simulink model "Verification_Decision_Module_w_History"  (R2015a)
settings: Solver=FixedStepDiscrete  StartTime=0.0  StopTime=10.0  FixedStep=delta_t  RelTol=1e-3
libraries: sldvlib x16
settings Model: Creator=Kerianne  LastModifiedBy=Kerianne
settings DataIOCC: SaveFormat=Structure
settings OptimizationCC: InlineParams=on  ExpressionDepthLimit=2147483647
settings DebuggingCC: UnderspecifiedInitializationDetection=Classic  MergeDetectMultiDrivingBlocksExec=none  SolverPrmCheckMsg=warning  StateNameClashWarn=warning
settings ConfigComp: Description=Design Verifier Custom Configuration Component  DVMaxTestCaseSteps=500  DVTestSuiteOptimization=CombinedObjectives (Nonlinear Extended)

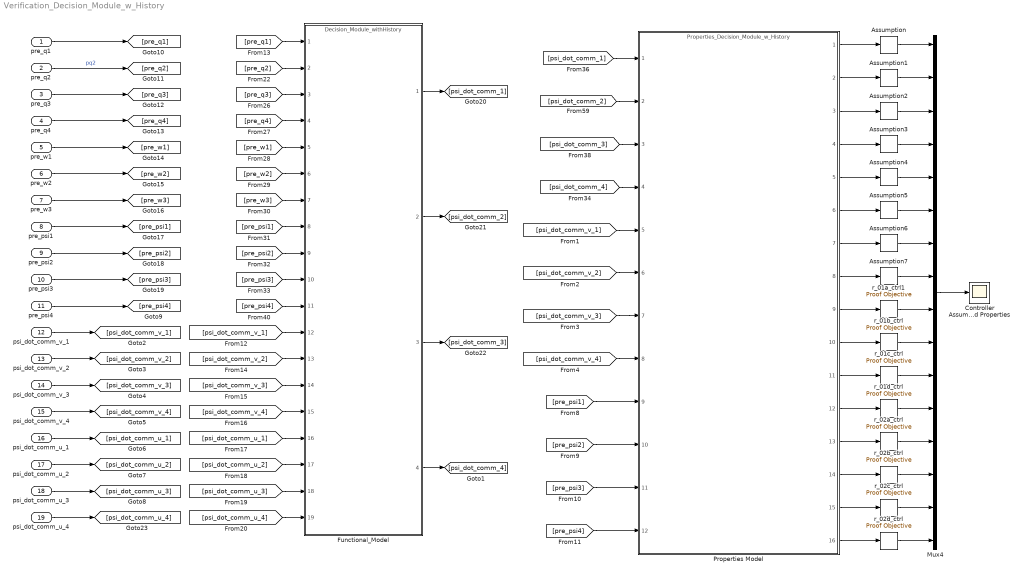
== system Verification_Decision_Module_w_History ==
  pre_q1 : Inport
  pre_q2 : Inport  Port=2
  pre_q3 : Inport  Port=3
  pre_q4 : Inport  Port=4
  pre_w1 : Inport  Port=5
  pre_w2 : Inport  Port=6
  pre_w3 : Inport  Port=7
  pre_psi1 : Inport  Port=8
  pre_psi2 : Inport  Port=9
  pre_psi3 : Inport  Port=10
  pre_psi4 : Inport  Port=11
  psi_dot_comm_v_1 : Inport  Port=12
  psi_dot_comm_v_2 : Inport  Port=13
  psi_dot_comm_v_3 : Inport  Port=14
  psi_dot_comm_v_4 : Inport  Port=15
  psi_dot_comm_u_1 : Inport  Port=16
  psi_dot_comm_u_2 : Inport  Port=17
  psi_dot_comm_u_3 : Inport  Port=18
  psi_dot_comm_u_4 : Inport  Port=19
  Assumption{,1..7} (8 alike) : sldvlib/Objectives and Constraints/Assumption  enabled=on  customAVTBlockType=Assumption  intervals=true  initial=off  dispValues=on  outEnabled=on
      settings: AttributesFormatString=%<intervals>
  Controller Assumptions and Properties : Scope
      settings: ShowLegends=on  YMin=-1  YMax=2
  Functional_Model : ModelReference  ModelNameDialog=Decision_Module_withHistory.slx  SimulationMode=Normal  ModelReferenceVersion=1.60  CopyOfModelName=Decision_Module_withHistory.slx  DefaultDataLogging=on
  Mux4 : Mux  Inputs=16
  Properties Model : ModelReference  ModelNameDialog=Properties_Decision_Module_w_History.slx  SimulationMode=Normal  ModelReferenceVersion=1.94  CopyOfModelName=Properties_Decision_Module_w_History.slx  DefaultDataLogging=on
  r_01a_ctrl1 : sldvlib/Objectives and Constraints/Proof Objective  Tag=g4  enabled=on  customAVTBlockType=Proof Objective  intervals=true  dispValues=on  outEnabled=on  enableStopSim=off
      settings: AttributesFormatString=%<intervals>
  r_01b_ctrl : sldvlib/Objectives and Constraints/Proof Objective  Tag=g4  enabled=on  customAVTBlockType=Proof Objective  intervals=true  dispValues=on  outEnabled=on  enableStopSim=off
      settings: AttributesFormatString=%<intervals>
  r_01c_ctrl : sldvlib/Objectives and Constraints/Proof Objective  Tag=g4  enabled=on  customAVTBlockType=Proof Objective  intervals=true  dispValues=on  outEnabled=on  enableStopSim=off
      settings: AttributesFormatString=%<intervals>
  r_01d_ctrl : sldvlib/Objectives and Constraints/Proof Objective  Tag=g4  enabled=on  customAVTBlockType=Proof Objective  intervals=true  dispValues=on  outEnabled=on  enableStopSim=off
      settings: AttributesFormatString=%<intervals>
  r_02a_ctrl : sldvlib/Objectives and Constraints/Proof Objective  Tag=g4  enabled=on  customAVTBlockType=Proof Objective  intervals=true  dispValues=on  outEnabled=on  enableStopSim=off
      settings: AttributesFormatString=%<intervals>
  r_02b_ctrl : sldvlib/Objectives and Constraints/Proof Objective  Tag=g4  enabled=on  customAVTBlockType=Proof Objective  intervals=true  dispValues=on  outEnabled=on  enableStopSim=off
      settings: AttributesFormatString=%<intervals>
  r_02c_ctrl : sldvlib/Objectives and Constraints/Proof Objective  Tag=g4  enabled=on  customAVTBlockType=Proof Objective  intervals=true  dispValues=on  outEnabled=on  enableStopSim=off
      settings: AttributesFormatString=%<intervals>
  r_02d_ctrl : sldvlib/Objectives and Constraints/Proof Objective  Tag=g4  enabled=on  customAVTBlockType=Proof Objective  intervals=true  dispValues=on  outEnabled=on  enableStopSim=off
      settings: AttributesFormatString=%<intervals>
  wires:
  Mux4/1 -> Controller Assumptions and Properties/1
  pre_q1/1 -> [pre_q1]
  pre_q2/1 -> [pre_q2]  "pq2"
  pre_q3/1 -> [pre_q3]
  pre_q4/1 -> [pre_q4]
  pre_w1/1 -> [pre_w1]
  pre_w2/1 -> [pre_w2]
  pre_w3/1 -> [pre_w3]
  pre_psi1/1 -> [pre_psi1]
  pre_psi2/1 -> [pre_psi2]
  pre_psi3/1 -> [pre_psi3]
  pre_psi4/1 -> [pre_psi4]
  [pre_q1] -> Functional_Model/1
  [pre_q2] -> Functional_Model/2
  [pre_q3] -> Functional_Model/3
  [pre_q4] -> Functional_Model/4
  [pre_w1] -> Functional_Model/5
  [pre_w2] -> Functional_Model/6
  [pre_w3] -> Functional_Model/7
  [pre_psi1] -> Functional_Model/8
  [pre_psi2] -> Functional_Model/9
  [pre_psi3] -> Functional_Model/10
  [pre_psi4] -> Functional_Model/11
  Functional_Model/4 -> [psi_dot_comm_4]
  Functional_Model/3 -> [psi_dot_comm_3]
  Functional_Model/2 -> [psi_dot_comm_2]
  Functional_Model/1 -> [psi_dot_comm_1]
  [psi_dot_comm_4] -> Properties Model/4
  [psi_dot_comm_3] -> Properties Model/3
  [psi_dot_comm_2] -> Properties Model/2
  [psi_dot_comm_1] -> Properties Model/1
  [pre_psi1] -> Properties Model/9
  [pre_psi2] -> Properties Model/10
  [pre_psi3] -> Properties Model/11
  [pre_psi4] -> Properties Model/12
  Assumption/1 -> Mux4/1
  Properties Model/1 -> Assumption/1
  Properties Model/4 -> Assumption3/1
  Properties Model/3 -> Assumption2/1
  Properties Model/2 -> Assumption1/1
  Assumption1/1 -> Mux4/2
  Assumption2/1 -> Mux4/3
  Assumption3/1 -> Mux4/4
  [psi_dot_comm_v_1] -> Functional_Model/12
  [psi_dot_comm_v_2] -> Functional_Model/13
  [psi_dot_comm_v_3] -> Functional_Model/14
  [psi_dot_comm_v_4] -> Functional_Model/15
  [psi_dot_comm_u_1] -> Functional_Model/16
  [psi_dot_comm_u_2] -> Functional_Model/17
  [psi_dot_comm_u_3] -> Functional_Model/18
  [psi_dot_comm_u_4] -> Functional_Model/19
  psi_dot_comm_u_4/1 -> [psi_dot_comm_u_4]
  psi_dot_comm_u_3/1 -> [psi_dot_comm_u_3]
  psi_dot_comm_u_2/1 -> [psi_dot_comm_u_2]
  psi_dot_comm_u_1/1 -> [psi_dot_comm_u_1]
  psi_dot_comm_v_4/1 -> [psi_dot_comm_v_4]
  psi_dot_comm_v_3/1 -> [psi_dot_comm_v_3]
  psi_dot_comm_v_2/1 -> [psi_dot_comm_v_2]
  psi_dot_comm_v_1/1 -> [psi_dot_comm_v_1]
  Properties Model/16 -> r_02d_ctrl/1
  Properties Model/15 -> r_02c_ctrl/1
  Properties Model/14 -> r_02b_ctrl/1
  Properties Model/13 -> r_02a_ctrl/1
  Properties Model/12 -> r_01d_ctrl/1
  Properties Model/11 -> r_01c_ctrl/1
  Properties Model/10 -> r_01b_ctrl/1
  Properties Model/9 -> r_01a_ctrl1/1
  r_01a_ctrl1/1 -> Mux4/9
  r_01b_ctrl/1 -> Mux4/10
  r_01c_ctrl/1 -> Mux4/11
  r_01d_ctrl/1 -> Mux4/12
  r_02a_ctrl/1 -> Mux4/13
  r_02b_ctrl/1 -> Mux4/14
  r_02c_ctrl/1 -> Mux4/15
  r_02d_ctrl/1 -> Mux4/16
  [psi_dot_comm_v_1] -> Properties Model/5
  [psi_dot_comm_v_2] -> Properties Model/6
  [psi_dot_comm_v_3] -> Properties Model/7
  [psi_dot_comm_v_4] -> Properties Model/8
  Properties Model/5 -> Assumption4/1
  Assumption4/1 -> Mux4/5
  Properties Model/6 -> Assumption5/1
  Assumption5/1 -> Mux4/6
  Properties Model/7 -> Assumption6/1
  Properties Model/8 -> Assumption7/1
  Assumption6/1 -> Mux4/7
  Assumption7/1 -> Mux4/8
